simulink model "RB_KAIROS_ImpControl_OpSpace_quat_2020b_safety"  (R2020b)
settings: Solver=ode4  StartTime=0.0  StopTime=t_end  FixedStep=Ts  RelTol=1e-3
values from neighbouring files (symbols this model uses):
  am = 0.3    [RB_KAIROS_ImpControl_OpSpace_quat_2020b_safety_main.m]
  am_r = 0.3    [RB_KAIROS_ImpControl_OpSpace_quat_2020b_safety_main.m]
  Kc = diag(50*ones(6,1))    [RB_KAIROS_ImpControl_OpSpace_quat_2020b_safety_main.m]
  Kp = 2*[400;400;400;400;0;0;0]    [RB_KAIROS_ImpControl_OpSpace_quat_2020b_safety_main.m]
  Kv = [1000;1000;1000;[300;300;300;300;300;300;300]]    [RB_KAIROS_ImpControl_OpSpace_quat_2020b_safety_main.m]
  model_sample_time = 0.001    [RB_KAIROS_ImpControl_OpSpace_quat_2020b_safety_main.m]
  q_dot_0 = zeros(10,1)    [RB_KAIROS_ImpControl_OpSpace_quat_2020b_safety_main.m]
  T_i = K    [RB_KAIROS_ImpControl_OpSpace_quat_2020b_safety_main.m]
  tau_ext = [0 0 0 0 0 0 0 0 0 0 0]    [RB_KAIROS_ImpControl_OpSpace_quat_2020b_safety_main.m]
  v_SMU = 10    [RB_KAIROS_ImpControl_OpSpace_quat_2020b_safety_main.m]
  vm = 0.5    [RB_KAIROS_ImpControl_OpSpace_quat_2020b_safety_main.m]
  vm_r = 0.5    [RB_KAIROS_ImpControl_OpSpace_quat_2020b_safety_main.m]
undefined symbols (not defined in the file or in its folder): DiscIntNeverNeededParam, magnitude, q_0, sigbuilder_block, T_f
libraries: simulink x4, utils x4, transformations_lib x3
(part 14 of 17)

== matlab function RB_KAIROS_ImpControl_OpSpace_quat_2020b_safety/CONTROLLER /Kinematics and Dynamics/Kinematics - error representation/MATLAB Function1 ==
  data: J input; t output
function t = fcn(J)

t = 0;
%you can use normc(J) to see if one column gets near 0 and by this you get
%directions that are singular
D = sqrt(det(J*J'));
if(D < 10e-2)
    t = 1;
    disp(J)
end

== matlab function RB_KAIROS_ImpControl_OpSpace_quat_2020b_safety/CONTROLLER /Kinematics and Dynamics/Kinematics - error representation/MATLAB Function2 ==
  data: R_D_W_aug input; vt output; x_dot_d input; x_ddot_d input; vt_dot output; x_err input; x_dot_err input
function [vt, vt_dot] = compute_vt(R_D_W_aug, x_dot_d, x_ddot_d, x_err, x_dot_err)
% This function is used to compute the vectors vt and vt_dot defined in Ott book in order
% to convert the equation of motion to an equivalent representation using
% error on the task variables

% INPUTS:
% - R_W_D_aug is an extension of the ROTATION MATRIX from world frame to 
%   desired frame: [R_W_D 0; 0 R_W_D], it is a 6x6 matrix
% - omega_d, p_dot_d, p_err, eps_err, omega_err are all quantities defined in
%   the world frame (or space frame) W.
S_omega_d = calc_skewsymm(x_dot_d(4:6));
S_alfa_d = calc_skewsymm(x_ddot_d(4:6));

a = [x_dot_d(1:3) + S_omega_d*(x_err(1:3));
                x_dot_d(4:6)];

vt = R_D_W_aug*a;

vt_dot = R_D_W_aug*(-augment_matrix(S_omega_d)*a + [x_ddot_d(1:3) + S_alfa_d*x_err(1:3) + S_omega_d*x_dot_err(1:3);
                                                                  x_ddot_d(4:6)]);

end 


function S = calc_skewsymm(v)

S = [0 -v(3) v(2);
    v(3) 0 -v(1);
    -v(2) v(1) 0];
end

function M_aug = augment_matrix(M)

M_aug = [M, zeros(3,3);
             zeros(3,3), M];
end

== matlab function RB_KAIROS_ImpControl_OpSpace_quat_2020b_safety/CONTROLLER /Kinematics and Dynamics/Kinematics - error representation/MATLAB Function3 ==
  data: R_W_D_aug input; J_x output; J_b input
function J_x   =compute_J_x(R_W_D_aug, J_b)
% This function is used to compute the matrix J_x defined in Ott book in order
% to convert the equation of motion to an equivalent representation using
% error on the task variables

% INPUTS:
% - R_W_D_aug is an extension of the ROTATION MATRIX from world frame to 
%   desired frame: [R_W_D 0; 0 R_W_D], it is a 6x6 matrix
% - J_b is the body Jacobian of the robot 

J_x = R_W_D_aug*J_b;

== matlab function RB_KAIROS_ImpControl_OpSpace_quat_2020b_safety/Trajectory Generator/Subsystem1/MATLAB Function ==
  data: u input; y output
function y = fcn(u)

y = rotm2eul(u, 'XYZ')';

== matlab function RB_KAIROS_ImpControl_OpSpace_quat_2020b_safety/CONTROLLER /Kinematics and Dynamics/Kinematics - error representation/Whole-Body Jacobian ==
  data: qv input; J output size=[6,10]; qa input
function J = get_J(qv,qa)
%GET_J
%    J = GET_J(qv,qa)

%    This function was generated by the Symbolic Math Toolbox version 8.6.
%    14-Feb-2023 10:02:51

phi = qv(3);

q1 = qa(1);
q2 = qa(2);
q3 = qa(3);
q4 = qa(4);
q5 = qa(5);
q6 = qa(6);
t2 = cos(phi);
t3 = cos(q1);
t4 = cos(q2);
t5 = cos(q3);
t6 = cos(q4);
t7 = cos(q5);
t8 = cos(q6);
t9 = sin(phi);
t10 = sin(q1);
t11 = sin(q2);
t12 = sin(q3);
t13 = sin(q4);
t14 = sin(q5);
t15 = sin(q6);
t16 = t3.*t5;
t17 = t4.*t6;
t18 = t3.*t12;
t19 = t5.*t10;
t20 = t4.*t13;
t21 = t10.*t12;
t22 = -t9;
t23 = t10.*t11.*t13;
t24 = t11.*t12.*t14;
t28 = t3.*t6.*t11;
t29 = t5.*t6.*t11;
t31 = t3.*t11.*t13;
t32 = t6.*t10.*t11;
t33 = t5.*t11.*t13;
t34 = t7.*t11.*t12;
t41 = t4.*(7.9e+1./2.5e+2);
t44 = t5.*t11.*(3.3e+1./4.0e+2);
t47 = t3.*t11.*(7.9e+1./2.5e+2);
t50 = t10.*t11.*(7.9e+1./2.5e+2);
t124 = t2.*1.224646799147353e-16;
t125 = t9.*1.224646799147353e-16;
t138 = t3.*t11.*3.869883885305636e-17;
t139 = t10.*t11.*3.869883885305636e-17;
t25 = t4.*t16;
t26 = t4.*t18;
t27 = t4.*t19;
t30 = t4.*t21;
t36 = -t29;
t38 = -t31;
t39 = -t32;
t40 = -t34;
t42 = t17.*(4.8e+1./1.25e+2);
t43 = t18.*(3.3e+1./4.0e+2);
t45 = t20.*(3.3e+1./4.0e+2);
t46 = t21.*(3.3e+1./4.0e+2);
t48 = -t44;
t52 = t23.*(3.3e+1./4.0e+2);
t55 = t17+t33;
t57 = t28.*(4.8e+1./1.25e+2);
t59 = t29.*(3.3e+1./4.0e+2);
t60 = t32.*(4.8e+1./1.25e+2);
t61 = t33.*(4.8e+1./1.25e+2);
t62 = t31.*(3.3e+1./4.0e+2);
t127 = t2+t125;
t130 = t22+t124;
t132 = t28.*4.702643708725836e-17;
t133 = t32.*4.702643708725836e-17;
t136 = t18.*1.010333609296566e-17;
t137 = t21.*1.010333609296566e-17;
t141 = -t138;
t144 = t31.*1.010333609296566e-17;
t145 = t23.*1.010333609296566e-17;
t35 = -t25;
t37 = -t30;
t49 = -t45;
t51 = -t46;
t53 = t18+t27;
t54 = t19+t26;
t56 = t25.*(3.3e+1./4.0e+2);
t58 = t27.*(3.3e+1./4.0e+2);
t63 = -t52;
t65 = -t57;
t66 = -t62;
t69 = t20+t36;
t72 = t8.*t55;
t85 = t15.*t55.*(1.1e+1./1.25e+2);
t135 = -t132;
t142 = t25.*1.010333609296566e-17;
t143 = t27.*1.010333609296566e-17;
t147 = -t145;
t64 = -t56;
t67 = t16+t37;
t68 = t21+t35;
t70 = t6.*t53;
t71 = t7.*t54;
t73 = t13.*t53;
t74 = t14.*t54;
t78 = t7.*t69;
t79 = -t72;
t82 = t14.*t69;
t91 = t72.*(1.07e+2./1.0e+3);
t146 = -t142;
t75 = t6.*t68;
t76 = t7.*t67;
t77 = -t71;
t80 = t13.*t68;
t81 = t14.*t67;
t84 = t70.*(3.3e+1./4.0e+2);
t86 = t73.*(4.8e+1./1.25e+2);
t89 = t23+t70;
t94 = -t91;
t96 = t39+t73;
t97 = t24+t78;
t101 = t40+t82;
t104 = -t8.*(t32-t73);
t110 = t15.*(t32-t73).*(-1.1e+1./1.25e+2);
t112 = t15.*(t32-t73).*(1.1e+1./1.25e+2);
t114 = t8.*(t32-t73).*(-1.07e+2./1.0e+3);
t149 = t73.*4.702643708725836e-17;
t152 = t70.*1.010333609296566e-17;
t159 = t15.*(t32-t73).*(-1.077689183249671e-17);
t162 = t15.*(t32-t73).*1.077689183249671e-17;
t164 = t8.*(t32-t73).*(-1.310372075087668e-17);
t83 = -t76;
t87 = -t84;
t88 = -t86;
t90 = t75.*(3.3e+1./4.0e+2);
t92 = t80.*(4.8e+1./1.25e+2);
t98 = t28+t80;
t99 = t7.*t89;
t100 = t14.*t89;
t102 = t38+t75;
t105 = t15.*t97;
t106 = -t7.*(t31-t75);
t107 = -t14.*(t31-t75);
t109 = t8.*t97.*(1.1e+1./1.25e+2);
t150 = -t149;
t151 = t80.*4.702643708725836e-17;
t154 = -t152;
t155 = t75.*1.010333609296566e-17;
t93 = -t90;
t95 = -t92;
t103 = t8.*t98;
t108 = t15.*t98.*(1.1e+1./1.25e+2);
t115 = t105.*(1.07e+2./1.0e+3);
t117 = t81+t99;
t118 = t74+t106;
t119 = t83+t100;
t120 = t79+t105;
t122 = t77+t107;
t153 = -t151;
t156 = -t155;
t158 = t15.*t98.*1.077689183249671e-17;
t111 = -t108;
t113 = t103.*(1.07e+2./1.0e+3);
t121 = t15.*t117;
t123 = t15.*t118;
t126 = t8.*t117.*(1.1e+1./1.25e+2);
t128 = t8.*t118.*(1.1e+1./1.25e+2);
t148 = t94+t115;
t161 = -t158;
t163 = t103.*1.310372075087668e-17;
t167 = t8.*t117.*1.077689183249671e-17;
t168 = t8.*t118.*1.077689183249671e-17;
t116 = -t113;
t129 = t121.*(1.07e+2./1.0e+3);
t131 = -t128;
t134 = t123.*(1.07e+2./1.0e+3);
t157 = t104+t121;
t160 = t103+t123;
t169 = t121.*1.310372075087668e-17;
t170 = t123.*1.310372075087668e-17;
t171 = t85+t109+t148;
t140 = -t134;
t165 = t114+t129;
t166 = t113+t134;
t172 = -t157.*(t91-t115);
t174 = -t160.*(t91-t115);
t177 = t98.*t171;
t178 = -t171.*(t32-t73);
t180 = t42+t49+t59+t61+t171;
t181 = -t171.*(t76-t100);
t182 = -t171.*(t71+t14.*(t31-t75));
t183 = t171.*(t76-t100);
t199 = -t11.*t12.*(t52-t60+t84+t86+t110-t126-t129+t8.*(t32-t73).*(1.07e+2./1.0e+3));
t200 = t11.*t12.*(t52-t60+t84+t86+t110-t126-t129+t8.*(t32-t73).*(1.07e+2./1.0e+3));
t173 = -t165.*(t72-t105);
t175 = -t166.*(t72-t105);
t176 = t165.*(t72-t105);
t179 = t166.*(t72-t105);
t184 = t48+t180;
t185 = t54.*t180;
t186 = t67.*t180;
t189 = t112+t126+t165;
t191 = t111+t128+t166;
t202 = -t11.*t12.*(t57+t66+t90+t92+t108+t116+t131+t140);
t203 = t11.*t12.*(t57+t66+t90+t92+t108+t116+t131+t140);
t210 = -t4.*(t51+t56+t57+t66+t90+t92+t108+t116+t131+t140);
t211 = t47+t51+t56+t57+t66+t90+t92+t108+t116+t131+t140;
t187 = t3.*t11.*t184;
t188 = t10.*t11.*t184;
t192 = t41+t184;
t193 = t55.*t189;
t194 = t55.*t191;
t195 = -t189.*(t34-t82);
t196 = -t191.*(t34-t82);
t197 = t191.*(t34-t82);
t198 = t60+t63+t87+t88+t189;
t201 = t62+t65+t93+t95+t191;
t206 = t172+t176;
t208 = t174+t179;
t216 = t186+t200;
t217 = t185+t203;
t220 = t133+t136+t139+t143+t147+t150+t154+t162+t164+t167+t169+t211+1.1e+1./4.0e+1;
t190 = -t188;
t204 = t43+t58+t198;
t207 = t46+t64+t201;
t212 = t178+t193;
t213 = t177+t194;
t214 = t183+t195;
t215 = t182+t197;
t219 = t187+t210;
t205 = t4.*t204;
t209 = t50+t204;
t218 = t190+t205;
t221 = t135+t137+t141+t144+t146+t153+t156+t161+t163+t168+t170+t209+3.1e+1./2.0e+2;
J = reshape([1.0,0.0,0.0,0.0,0.0,0.0,0.0,1.0,0.0,0.0,0.0,0.0,t2.*t221+t9.*t220,-t2.*t220+t9.*t221,0.0,0.0,0.0,1.0,t127.*t209-t130.*t211,-t127.*t211-t130.*t209,0.0,0.0,0.0,1.0,-t3.*t127.*t192-t10.*t130.*t192,t3.*t130.*t192-t10.*t127.*t192,-t3.*t211-t10.*t209,-t3.*t130+t10.*t127,-t3.*t127-t10.*t130,0.0,t130.*t219-t127.*(t188-t205),t127.*t219+t130.*(t188-t205),-t10.*t11.*(t51+t56+t57+t66+t90+t92+t108+t116+t131+t140)+t3.*t11.*t204,-t3.*t11.*t127-t10.*t11.*t130,t3.*t11.*t130-t10.*t11.*t127,t4,t127.*t216+t130.*t217,t127.*t217-t130.*t216,t67.*(t57+t66+t90+t92+t108+t116+t131+t140)-t54.*(t52-t60+t84+t86+t110-t126-t129+t8.*(t32-t73).*(1.07e+2./1.0e+3)),-t54.*t127+t67.*t130,t54.*t130+t67.*t127,-t11.*t12,t127.*(t193-t171.*(t32-t73))+t130.*t213,-t130.*(t193-t171.*(t32-t73))+t127.*t213,t98.*t189+t191.*(t32-t73),-t98.*t127-t130.*(t32-t73),t98.*t130-t127.*(t32-t73),t55,t127.*t214+t130.*(t196+t171.*(t71+t14.*(t31-t75))),-t130.*t214+t127.*(t196+t171.*(t71+t14.*(t31-t75))),t189.*(t71+t14.*(t31-t75))-t191.*(t76-t100),-t127.*(t71+t14.*(t31-t75))+t130.*(t76-t100),t130.*(t71+t14.*(t31-t75))+t127.*(t76-t100),t101,-t127.*t206-t130.*t208,-t127.*t208+t130.*t206,t157.*t166-t160.*t165,t127.*t160-t130.*t157,-t127.*t157-t130.*t160,t120],[6,10]);

== matlab function RB_KAIROS_ImpControl_OpSpace_quat_2020b_safety/CONTROLLER /MATLAB Function ==
  data: qa_des input; qa_des_new output; qv input
function qa_des_new = fcn(qa_des,qv)

qa_des_new = qa_des;
% qa_des_new(1) = qa_des_new(1)+qv(3);

== matlab function RB_KAIROS_ImpControl_OpSpace_quat_2020b_safety/CONTROLLER /Primary task - Controller/MATLAB Function ==
  data: Kc input; Dc output; Lambda input
function Dc = compute_damping(Kc,Lambda)
%  COMPUTE_DAMPING Computes damping matrix to enforce desired second order
%  system behaviour.
%
%   Dc = COMPUTE_DAMPING(Kc,Lambda) computes the damping depending on 
%        stiffness matrix Kc (which has to be constant for stability) and
%        inertia matrix Lambda (which is time varying since no inertia 
%        shaping is applied).
%   
%   Reference: Cartesian Impedance Control of Redundant and Flexible-Joint
%              Robots, C. Ott 2005, page 36-37.
%   See also EIG

% % DAMPING MATRIX (varying) simplified
zeta = 1*ones(6,1);

A = real(sqrtm(Lambda));
Kc_1 = real(sqrtm(Kc));
D0 = diag(zeta);
Dc = A*D0*Kc_1 + Kc_1*D0*A;

% % DAMPING MATRIX (varying)
% %Generalized eigenvalue decomposition for the pair (Kc,Lambda)
% [eigvecs,eigvals] = eig(Kc, Lambda);
% eigvals = real(eigvals);
% eigvecs = real(eigvecs);
% %sorting eigs by magnitude
% %[eigvals,sidx] = sort(diag(eigvals),'descend');
% 
% %Finding matrices that satisfy K = Q'K0Q and Lambda = Q'*Q
% K0 = eigvals;
% %V = eigvecs(:,sidx);
% Q_T = Lambda*eigvecs;
% Q = Q_T';
% 
% %Damping matrix computation
% zeta = 1*ones(6,1); %Imposing an overdamped behaviour
% D0 = diag(zeta).*K0;
% Dc = 2*Q_T*D0*Q;
% 
%OLD implementation where stiffness and damping were retrieven from
%configuration parameters
%function [Kc,Dc] = compute_stiffness_damping(J, J_T, J_i, J_d, Lambda)

% Kq_veh = [750*ones(2,1); 750]; 
% Dq_veh = [800;800;800];
% Kq_arm = [350;250;100;170;50;20;10];
% Dq_arm = [60;200;120;150;20;30;5];
% 
% Kq = diag([Kq_veh;Kq_arm]);
% Dq = diag([Dq_veh;Dq_arm]);
% 
% Dc = J_i'*Dq*J_i;
% Kc = J_i'*(Kq-J_T*Dc*J_d)*J_i;

% Kc = diag([150;180;105;1.5;15;52.5]);
% Dc = diag([180;200;80;10;10;6]);

== matlab function RB_KAIROS_ImpControl_OpSpace_quat_2020b_safety/CONTROLLER /Secondary task - Controller/MATLAB Function ==
  data: qa_des input; qa input; tau_n output; qa_dot input; qv_dot input; M input; J_x_T input; J_x_i input; Kp input; Kv input
function tau_n = compute_null_space_torque(qa_des, qa, qa_dot, qv_dot, M, J_x_T, J_x_i, Kp, Kv)


%% Version 1: Try to keep the robot joints in their mid position
% q_max = [2.3093; 1.5133; 2.4937; -0.4461; 2.4800; 4.2094; 2.6895];
% q_min = [-2.3093; -1.5133; -2.4937; -2.7478; -2.4800; 0.8521; -2.6895];
% tau_0 = -M*[Kv(1:3).*qv_dot;2*Kp.*(qa-(q_max+q_min)./2)+Kv(4:10).*qa_dot];
% Good but the mid config. of every joint is not super good for any motion

%% Version 2: Mantain a certain configuration 
%Compute generalized joint torque based on the gradient of the potential
%that is used to mantain a certain configuration of the arm.

    tau_0 = -M*[Kv(1:3).*qv_dot;
         Kp.*(qa-qa_des)+Kv(4:10).*qa_dot]; 
    

%% Projection of the torque in the null space
tau_n = (eye(size(M,2))-J_x_T*J_x_i')*tau_0;

== matlab function RB_KAIROS_ImpControl_OpSpace_quat_2020b_safety/EE to task space quaternion quantities/Augment matrix ==
  data: R_W_D input; R_D_W_aug output
function R_D_W_aug = augment_matrix(R_W_D)

R_D_W_aug = [R_W_D', zeros(3,3);
             zeros(3,3), R_W_D'];

== matlab function RB_KAIROS_ImpControl_OpSpace_quat_2020b_safety/EE to task space quaternion quantities/Get Pose in quaternions ==
  data: T_W_EE input; p_EE output; qt_EE output
function [p_EE, qt_EE] = tform2pose_quat(T_W_EE)
% Retrieves the pose of the end effector using quaternion representation
% for the orientation 

p_EE = T_W_EE(1:3,4);
qt_EE = tform2quat(T_W_EE)';

== matlab function RB_KAIROS_ImpControl_OpSpace_quat_2020b_safety/EE to task space quaternion quantities/MATLAB Function ==
  data: qt input; qt_unit output
function qt_unit = qt_norm(qt)

qt_unit = qt./norm(qt);

== matlab function RB_KAIROS_ImpControl_OpSpace_quat_2020b_safety/EE to task space quaternion quantities/MATLAB Function1 ==
  data: R input; qt output
function qt = rotm2quat(R)

qt = rotm2quat(R)';
